simulink model "SensorTest"  (R2017b)
settings: Solver=VariableStepAuto  StartTime=0.0  StopTime=inf  RelTol=1e-3
settings Model: Creator=SYSTEM  LastModifiedBy=segadiallo
settings HardwareCC: ProdBitPerLong=64  ProdHWDeviceType=Intel->x86-64 (Mac OS X)
settings CodeAppCC: StateflowObjectComments=on

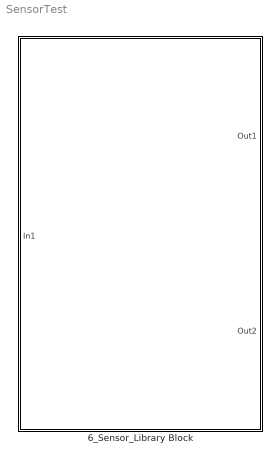
== system SensorTest ==
  6_Sensor_Library Block : Subsystem
      mask help: IR Sensor Test
      mask Display:
      | disp('6_Sensors_Test')
      | port_label('output',1,'Status')
      | port_label('output',2,'display')
      | port_label('input',1,'InputV')

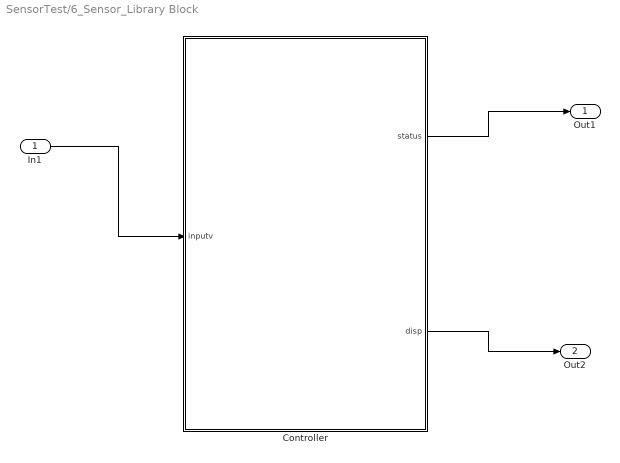
== system SensorTest/6_Sensor_Library Block ==
  In1 : Inport
  Controller : Stateflow chart  TreatAsAtomicUnit=on
  Out1 : Outport
  Out2 : Outport  Port=2
  wires:
  In1/1 -> Controller/1(inputv)
  Controller/1(status) -> Out1/1
  Controller/2(disp) -> Out2/1

== stateflow chart SensorTest/6_Sensor_Library Block/Controller ==
  state init
    entry:
    coder.extrinsic('evalin');
    obj = evalin('base','objWs');
    disp=[0;0;0;0;0;0];
    status = 0
  state NoCommand
    entry:
    disp=[0;0;0;0;0;0];
    status=0
  state Start
    entry:
    du:
    coder.extrinsic('evalin');
    obj = evalin('base','objWs');
    coder.extrinsic('RangeStateRoomba')
    disp=RangeStateRoomba(obj);
    status = 1;
  (default) -> NoCommand
  NoCommand -> init : after(0.5,sec)
  init -> Start : [inputv==3]
  Start -> init [order 2] : [inputv==1]
  Start -> Start [order 1] : after(0.1,sec)
  data: inputv input size=1; status output; so local; disp output double size=6; obj local
